simulink model "fixpt_constant"  (R2015b)
settings: Solver=FixedStepDiscrete  StartTime=0.0  StopTime=0  FixedStep=1  RelTol=1e-3
settings Model: Creator=y_yama  LastModifiedBy=amatsumo
settings DataIOCC: SaveFormat=Array  SignalLoggingSaveFormat=ModelDataLogs  SaveOutput=off  SignalLogging=off  SaveTime=off
settings OptimizationCC: DefaultParameterBehavior=Inlined  InlineInvariantSignals=on  ExpressionDepthLimit=2147483647  ZeroExternalMemoryAtStartup=off  ZeroInternalMemoryAtStartup=off  InitFltsAndDblsToZero=on  NoFixptDivByZeroProtection=on  EfficientFloat2IntCast=on  OptimizeModelRefInitCode=on  LifeSpan=1
settings DebuggingCC: UnderspecifiedInitializationDetection=Classic  MergeDetectMultiDrivingBlocksExec=none  SolverPrmCheckMsg=warning  InheritedTsInSrcMsg=none  FcnCallInpInsideContextMsg=UseLocalSettings  StateNameClashWarn=warning
settings HardwareCC: ProdBitPerPointer=32  ProdLargestAtomicFloat=None  ProdWordSize=32  ProdHWDeviceType=Generic->32-bit Embedded Processor
settings RTWCC: SystemTargetFile=ert.tlc  GenCodeOnly=on  TemplateMakefile=ert_default_tmf  Description=Real-Time Workshop Embedded Coder (no auto configuration)  GenerateReport=on  IncludeHyperlinkInReport=on  LaunchReport=on
settings CodeAppCC: GenerateComments=off  IgnoreCustomStorageClasses=off  CustomSymbolStrGlobalVar=$N$M  CustomSymbolStrType=$N$R$M  SimulinkBlockComments=off  InternalIdentifier=Classic
settings ERTTargetCC: GenerateSampleERTMain=on  IncludeMdlTerminateFcn=off  SuppressErrorStatus=on  SupportAbsoluteTime=off  SupportNonFinite=off  SupportComplex=off  InlinedParameterPlacement=NonHierarchical  ERTCustomFileTemplate=example_file_process.tlc
settings ConfigComp: CovModelRefEnable=Off  CovSFcnEnable=off

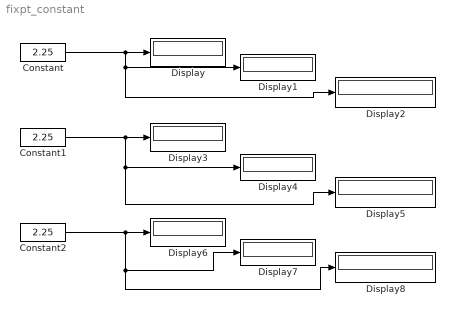
== system fixpt_constant ==
  Constant : Constant  Value=2.25  OutDataTypeStr=fixdt(1,8,0)  SampleTime=-1
      settings: AttributesFormatString=DataType = %<OutDataTypeStr>
  Constant1 : Constant  Value=2.25  OutDataTypeStr=fixdt(1,8,1)  SampleTime=-1
      settings: AttributesFormatString=DataType = %<OutDataTypeStr>
  Constant2 : Constant  Value=2.25  OutDataTypeStr=fixdt(1,8,2)  SampleTime=-1
      settings: AttributesFormatString=DataType = %<OutDataTypeStr>
  Display{,1..8} (9 alike) : Display
      Display settings: AttributesFormatString=Format = %<Format>
      Display1 settings: AttributesFormatString=Format = %<Format>  Format=hex (Stored Integer)
      Display2 settings: AttributesFormatString=Format = %<Format>  Format=binary (Stored Integer)
      Display3 settings: AttributesFormatString=Format = %<Format>
      Display4 settings: AttributesFormatString=Format = %<Format>  Format=hex (Stored Integer)
      Display5 settings: AttributesFormatString=Format = %<Format>  Format=binary (Stored Integer)
      Display6 settings: AttributesFormatString=Format = %<Format>
      Display7 settings: AttributesFormatString=Format = %<Format>  Format=hex (Stored Integer)
      Display8 settings: AttributesFormatString=Format = %<Format>  Format=binary (Stored Integer)
  wires:
  Constant/1 -> Display/1, Display1/1, Display2/1
  Constant1/1 -> Display5/1, Display4/1, Display3/1
  Constant2/1 -> Display8/1, Display7/1, Display6/1
